simulink model "Project_sim"  (R2025b)
settings: Solver=ode4  StartTime=0.0  StopTime=2*T  FixedStep=0.1  RelTol=1e-3
values from neighbouring files (symbols this model uses):
  a = 3000+R_E    [RUN_ME.m]
  A_0 = [cos(th0+epsilon1) sin(th0+epsilon1) 0; -sin(th0+epsilon1) cos(th0+epsilon1) 0; 0 0 1]*    [1 0 0; 0 cos(i+epsilon2) sin(i+epsilon2); 0 -sin(i+epsilon2) cos(i+epsilon2)]    [RUN_ME.m]
  alpha1 = 0.72    [RUN_ME.m]
  alpha_G0 = 0    [RUN_ME.m]
  AU = astroConstants(2)    [RUN_ME.m]
  b_gyro = deg2rad(0.01*rand(1))    [RUN_ME.m]
  b_mag = 15e-9    (= 1.5e-08)    [RUN_ME.m]
  b_sun = deg2rad(0.1*rand(1))    [RUN_ME.m]
  c_time = 100    [RUN_ME.m]
  D = zeros(3)    [RUN_ME.m]
  den_cz_mag = double(sym2poly(den8_z_mag))    [RUN_ME.m]
  den_cz_sun = double(sym2poly(den8_z_sun))    [RUN_ME.m]
  e = 0.2    [RUN_ME.m]
  epsilon = astroConstants(8)    [RUN_ME.m]
  g_IGRF = [ ... (first row only)    [RUN_ME.m]
  gyro_delay = 1    [RUN_ME.m]
  gyro_mounting = eye(3)    [RUN_ME.m]
  h_IGRF = [ ... (first row only)    [RUN_ME.m]
  I = [Ix 0 0; 0 Iy 0; 0 0 Iz]    [RUN_ME.m]
  i = deg2rad(30)    [RUN_ME.m]
  j_B = [0.01; 0.05; 0.01]    [RUN_ME.m]
  K = place(A, -B, a_controlled)    [RUN_ME.m]
  k1 = 20e-4    (= 0.002)    [RUN_ME.m]
  k1_tilde = 5e-4    (= 0.0005)    [RUN_ME.m]
  k2 = 2e-4    (= 0.0002)    [RUN_ME.m]
  Mis_gyro = deg2rad(0.1*rand(3,1))    [RUN_ME.m]
  Mis_mag = deg2rad(0.1*rand(3,1))    [RUN_ME.m]
  Mis_sun = deg2rad(0.1*rand(3,1))    [RUN_ME.m]
  mu = astroConstants(13)    [RUN_ME.m]
  n = sqrt(mu/a^3)    [RUN_ME.m]
  noise_density_mag = 16e-9    (= 1.6e-08)    [RUN_ME.m]
  Nonorthog_err_gyro = deg2rad(0.1*rand(3,1))    [RUN_ME.m]
  Nonorthog_err_mag = deg2rad(1)*ones(3,1)    [RUN_ME.m]
  num_cz_mag = double(sym2poly(num8_z_mag))    [RUN_ME.m]
  num_cz_sun = double(sym2poly(num8_z_sun))    [RUN_ME.m]
  R_E = astroConstants(23)    [RUN_ME.m]
  R_sun = astroConstants(3)    [RUN_ME.m]
  saturation_gyro = deg2rad(100)    [RUN_ME.m]
  saturation_mag = 60e-6    (= 6e-05)    [RUN_ME.m]
  SF = deg2rad(20*5.25e-3)    [RUN_ME.m]
  SFn = 0.02/100    (= 0.0002)    [RUN_ME.m]
  sigma_ARW = ARW/sqrt(Ts_gyro)    [RUN_ME.m]
  sigma_bias = bias_instability/sqrt(Ts_gyro)    [RUN_ME.m]
  sigma_RRW = RRW/sqrt(Ts_gyro)    [RUN_ME.m]
  sigma_sun = deg2rad(0.5)    [RUN_ME.m]
  th0 = deg2rad(0)    [RUN_ME.m]
  Ts = 0.1    [RUN_ME.m]
  Ts_gyro = 0.1    [RUN_ME.m]
  Ts_mag = 0.1    [RUN_ME.m]
  Ts_sun = 0.1    [RUN_ME.m]
  w_E = 2*pi/T_E    [RUN_ME.m]
  wx_0 = rand(1)*pi/6    [RUN_ME.m]
  wy_0 = rand(1)*pi/6    [RUN_ME.m]
  wz_0 = rand(1)*pi/6    [RUN_ME.m]
undefined symbols (not defined in the file or in its folder): DiscIntNeverNeededParam, dspblkCoreblockFVToolHelper, gcbh, magnitude, precision_sun, RW
libraries: Lib_rotation_matrix x17, matrix_library x11, simulink x3
(part 2 of 3)

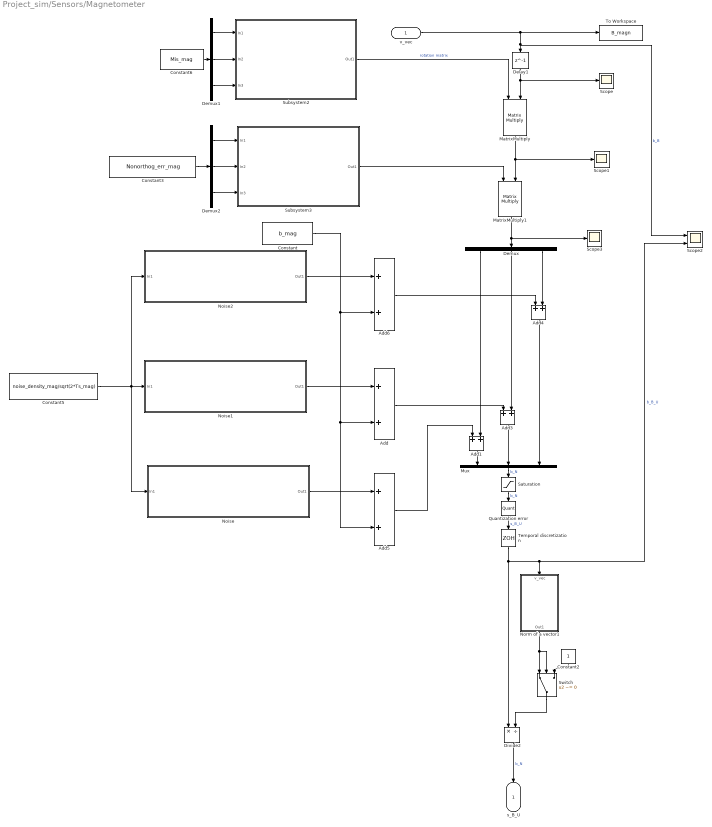
== system Project_sim/Sensors/Magnetometer ==
  v_vec : Inport
  Add{,1,3..6} (6 alike) : Sum
  Constant : Constant  Value=b_mag
  Constant2 : Constant
  Constant3 : Constant  Value=Nonorthog_err_mag
  Constant5 : Constant  Value=noise_density_mag/sqrt(2*Ts_mag)
  Constant6 : Constant  Value=Mis_mag
  Delay1 : Delay  DelayLength=1
  Demux : Demux  Outputs=3
  Demux1 : Demux  Outputs=3
  Demux2 : Demux  Outputs=3
  Divide2 : Product  Inputs=*/
  MatrixMultiply : Product  Multiplication=Matrix(*)
  MatrixMultiply1 : Product  Multiplication=Matrix(*)
  Mux : Mux  Inputs=3
  Noise : Subsystem
  Noise1 : Subsystem
  Noise2 : Subsystem
  Norm of a vector1 : Subsystem
  Quantization error : Quantizer  QuantizationInterval=precision_mag
  Saturation : Saturate  UpperLimit=saturation_mag  LowerLimit=-saturation_mag
  Scope : Scope
      settings: DataLoggingVariableName=ScopeData11  DataLoggingSaveFormat=Array
  Scope1 : Scope
      settings: DataLoggingVariableName=ScopeData13  DataLoggingSaveFormat=Array
  Scope2 : Scope  NumInputPorts=2
      settings: DataLoggingVariableName=ScopeData12  DataLoggingSaveFormat=Array
  Scope3 : Scope
      settings: DataLoggingVariableName=ScopeData15  DataLoggingSaveFormat=Array
  Subsystem2 : Subsystem
  Subsystem3 : Subsystem
  Switch : Switch  Criteria=u2 ~= 0  SaturateOnIntegerOverflow=off  InputSameDT=off
  Temporal discretization : ZeroOrderHold  SampleTime=Ts_mag
  To Workspace : ToWorkspace  VariableName=B_magn  SampleTime=-1
  s_B_U : Outport
  wires:
  v_vec/1 -> Scope2/1, Delay1/1, To Workspace/1  "b_B"
  Subsystem2/1(Out1) -> MatrixMultiply/1  "rotation matrix"
  Norm of a vector1/1(Out1) -> Switch/2, Switch/1
  Demux/1 -> Add1/2
  Demux/2 -> Add3/2
  Demux/3 -> Add4/2
  Add1/1 -> Mux/1
  Add3/1 -> Mux/2
  Add4/1 -> Mux/3
  Constant5/1 -> Noise2/1(In1), Noise/1(In1), Noise1/1(In1)
  Noise/1(Out1) -> Add5/1
  Noise1/1(Out1) -> Add/1
  Noise2/1(Out1) -> Add6/1
  Constant/1 -> Add5/2, Add/2, Add6/2
  Add6/1 -> Add4/1
  Add/1 -> Add3/1
  Add5/1 -> Add1/1
  Demux1/2 -> Subsystem2/2(In2)
  Constant6/1 -> Demux1/1
  Demux1/3 -> Subsystem2/3(In3)
  Demux1/1 -> Subsystem2/1(In1)
  Demux2/2 -> Subsystem3/2(In2)
  Constant3/1 -> Demux2/1
  Demux2/3 -> Subsystem3/3(In3)
  Subsystem3/1(Out1) -> MatrixMultiply1/1
  Demux2/1 -> Subsystem3/1(In1)
  Divide2/1 -> s_B_U/1  "b_N"
  Mux/1 -> Saturation/1  "b_N"
  Saturation/1 -> Quantization error/1  "b_N"
  Switch/1 -> Divide2/2
  Constant2/1 -> Switch/3
  Delay1/1 -> Scope/1, MatrixMultiply/2
  MatrixMultiply/1 -> Scope1/1, MatrixMultiply1/2
  MatrixMultiply1/1 -> Scope3/1, Demux/1
  Quantization error/1 -> Temporal discretization/1  "s_B_U"
  Temporal discretization/1 -> Scope2/2, Norm of a vector1/1(v_vec), Divide2/1  "b_B_U"

== system Project_sim/Sensors/Sun sensor ==
  In1 : Inport
  Enable : EnablePort  StatesWhenEnabling=reset
  Add1 : Sum
  Add3 : Sum
  Add4 : Sum
  Constant : Constant  Value=b_sun
  Constant1 : Constant  Value=Mis_sun
  Constant2 : Constant  Value=sigma_sun
  Delay1 : Delay  DelayLength=1
  Demux : Demux  Outputs=3
  Matrix Multiply1 : Product  Multiplication=Matrix(*)
  Matrix Multiply2 : Product  Multiplication=Matrix(*)
  Noise : Subsystem
  Noise1 : Subsystem
  Noise2 : Subsystem
  Precision : Subsystem  Commented=on
  Scope : Scope
      settings: DataLoggingVariableName=ScopeData6  DataLoggingSaveFormat=Array
  Subsystem1 : Subsystem
  Subsystem2 : Subsystem
  Temporal discretization : ZeroOrderHold  SampleTime=Ts_sun
  s_B_U : Outport  OutputWhenDisabled=reset  InitialOutput=-2
  wires:
  Temporal discretization/1 -> Scope/1, s_B_U/1  "s_B_U"
  In1/1 -> Delay1/1  "s_B"
  Subsystem1/1(Out1) -> Matrix Multiply1/1
  Subsystem2/1(Out1) -> Matrix Multiply2/1
  Matrix Multiply2/1 -> Matrix Multiply1/2
  Noise/1(Out1) -> Add1/2
  Constant1/1 -> Demux/1
  Demux/1 -> Subsystem2/1(In1)
  Demux/3 -> Subsystem2/3(In3)
  Demux/2 -> Subsystem2/2(In2)
  Noise1/1(Out1) -> Add3/2
  Add3/1 -> Subsystem1/3(In3)  "scale factor"
  Noise2/1(Out1) -> Add4/2
  Constant2/1 -> Noise1/1(In1), Noise/1(In1), Noise2/1(In1)
  Constant/1 -> Add3/1, Add1/1, Add4/1
  Add1/1 -> Subsystem1/2(In2)  "scale factor"
  Add4/1 -> Subsystem1/1(In1)  "scale factor"
  Delay1/1 -> Matrix Multiply2/2
  Matrix Multiply1/1 -> Temporal discretization/1

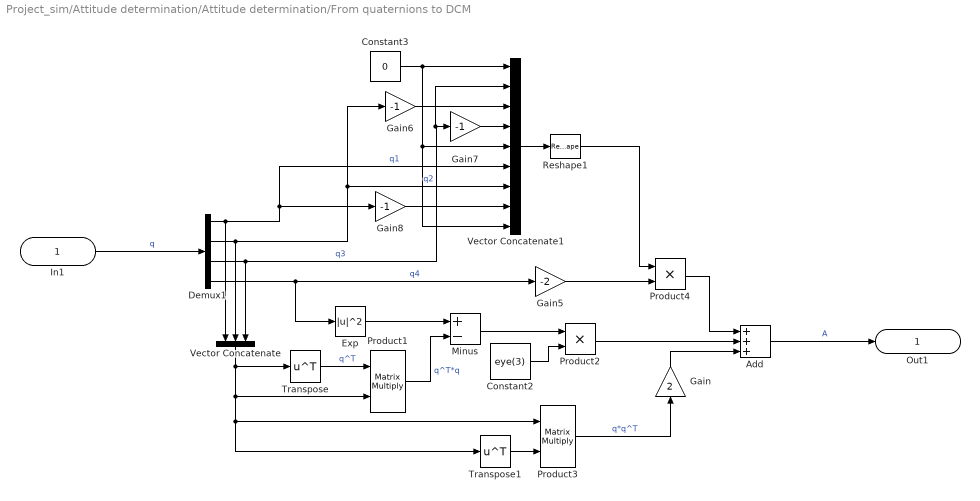
== system Project_sim/Attitude determination/Attitude determination/From quaternions to DCM ==
  In1 : Inport
  Add : Sum  Inputs=+++
  Constant2 : Constant  Value=eye(3)
  Constant3 : Constant  Value=0
  Demux1 : Demux
  Exp : Math  Operator=magnitude^2
  Gain : Gain  Gain=2
  Gain5 : Gain  Gain=-2
  Gain6 : Gain  Gain=-1
  Gain7 : Gain  Gain=-1
  Gain8 : Gain  Gain=-1
  Minus : Sum  Inputs=+-
  Product1 : Product  Multiplication=Matrix(*)
  Product2 : Product
  Product3 : Product  Multiplication=Matrix(*)
  Product4 : Product
  Reshape1 : Reshape  OutputDimensionality=Customize  OutputDimensions=[3,3]
  Transpose : Math  Operator=transpose
  Transpose1 : Math  Operator=transpose
  Vector Concatenate : Concatenate  NumInputs=3
  Vector Concatenate1 : Concatenate  NumInputs=9
  Out1 : Outport
  wires:
  Constant2/1 -> Product2/2
  Transpose1/1 -> Product3/2
  Exp/1 -> Minus/1
  Product2/1 -> Add/2
  Vector Concatenate/1 -> Product1/2, Product3/1, Transpose1/1, Transpose/1
  Transpose/1 -> Product1/1  "q^T"
  Gain/1 -> Add/3
  Add/1 -> Out1/1  "A"
  Demux1/4 -> Exp/1, Gain5/1  "q4"
  Demux1/1 -> Vector Concatenate/1, Gain8/1, Vector Concatenate1/6  "q1"
  Vector Concatenate1/1 -> Reshape1/1
  Product1/1 -> Minus/2  "q^T*q"
  Gain5/1 -> Product4/2
  In1/1 -> Demux1/1  "q"
  Minus/1 -> Product2/1
  Demux1/2 -> Vector Concatenate1/7, Gain6/1, Vector Concatenate/2  "q2"
  Gain8/1 -> Vector Concatenate1/8
  Product4/1 -> Add/1
  Reshape1/1 -> Product4/1
  Constant3/1 -> Vector Concatenate1/9, Vector Concatenate1/5, Vector Concatenate1/1
  Demux1/3 -> Vector Concatenate1/2, Gain7/1, Vector Concatenate/3  "q3"
  Gain6/1 -> Vector Concatenate1/3
  Gain7/1 -> Vector Concatenate1/4
  Product3/1 -> Gain/1  "q*q^T"

== system Project_sim/Attitude determination/Attitude determination/Trace of a matrix ==
  M : Inport
  Add2 : Sum  Inputs=+++
  Demux : Demux  Outputs=9
  Reshape : Reshape  OutputDimensionality=Column vector (2-D)
  tr(M) : Outport
  wires:
  Demux/5 -> Add2/2
  Demux/1 -> Add2/1
  Reshape/1 -> Demux/1
  Demux/9 -> Add2/3
  M/1 -> Reshape/1
  Add2/1 -> tr(M)/1  "tr(M)"

== system Project_sim/Control system/Control Manager/If Action Subsystem ==
  In1 : Inport
  Action Port : ActionPort  InitializeStates=reset  PropagateVarSize=During execution  ActionPortLabel=if(u1<u2 & u3 >100)
  Out1 : Outport
  wires:
  In1/1 -> Out1/1  "1"

== system Project_sim/Control system/Control Manager/If Action Subsystem1 ==
  In1 : Inport
  Action Port : ActionPort  InitializeStates=reset  PropagateVarSize=During execution  ActionPortLabel=if(u1 ==1 & u2 < u3 & u4 <u5 & u6 > 200)
  Out1 : Outport
  wires:
  In1/1 -> Out1/1  "1"

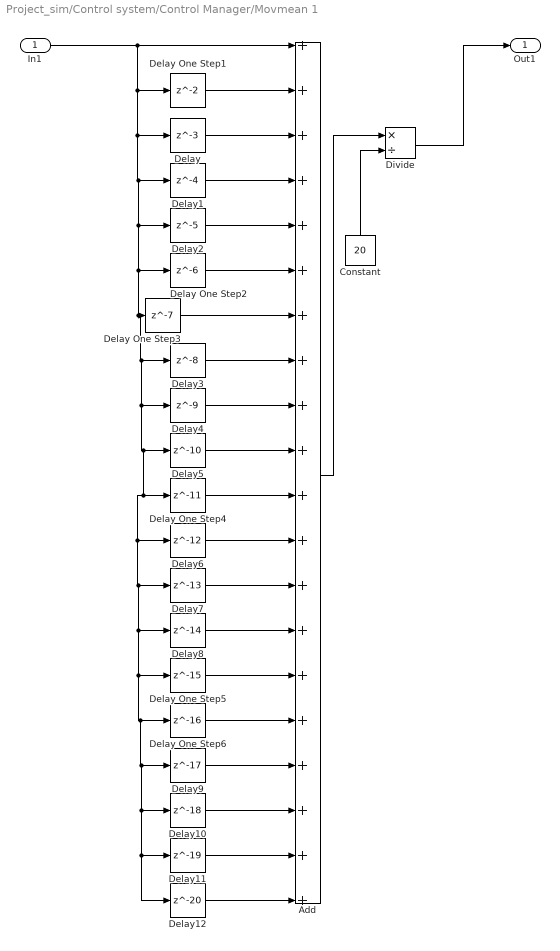
== system Project_sim/Control system/Control Manager/Movmean 1 ==
  In1 : Inport
  Add : Sum  Inputs=++++++++++++++++++++
  Constant : Constant  Value=20
  Delay : Delay  DelayLength=3
  Delay One Step1 : Delay
  Delay One Step2 : Delay  DelayLength=6
  Delay One Step3 : Delay  DelayLength=7
  Delay One Step4 : Delay  DelayLength=11
  Delay One Step5 : Delay  DelayLength=15
  Delay One Step6 : Delay  DelayLength=16
  Delay1 : Delay  DelayLength=4
  Delay10 : Delay  DelayLength=18
  Delay11 : Delay  DelayLength=19
  Delay12 : Delay  DelayLength=20
  Delay2 : Delay  DelayLength=5
  Delay3 : Delay  DelayLength=8
  Delay4 : Delay  DelayLength=9
  Delay5 : Delay  DelayLength=10
  Delay6 : Delay  DelayLength=12
  Delay7 : Delay  DelayLength=13
  Delay8 : Delay  DelayLength=14
  Delay9 : Delay  DelayLength=17
  Divide : Product  Inputs=*/
  Out1 : Outport
  wires:
  Delay One Step1/1 -> Add/2
  Delay/1 -> Add/3
  Delay1/1 -> Add/4
  Delay2/1 -> Add/5
  Add/1 -> Divide/1
  Constant/1 -> Divide/2
  Divide/1 -> Out1/1
  Delay One Step2/1 -> Add/6
  Delay One Step3/1 -> Add/7
  Delay3/1 -> Add/8
  Delay4/1 -> Add/9
  Delay5/1 -> Add/10
  Delay One Step6/1 -> Add/16
  Delay6/1 -> Add/12
  Delay10/1 -> Add/18
  Delay11/1 -> Add/19
  Delay One Step5/1 -> Add/15
  Delay7/1 -> Add/13
  Delay9/1 -> Add/17
  Delay8/1 -> Add/14
  In1/1 -> Delay2/1, Delay One Step2/1, Delay8/1, Delay One Step5/1, Delay12/1, Delay11/1, Delay10/1, Delay9/1, Delay One Step6/1, Delay7/1, Delay6/1, Delay One Step4/1, Delay5/1, Delay4/1, Delay3/1, Delay One Step3/1, Delay1/1, Delay/1, Delay One Step1/1, Add/1
  Delay One Step4/1 -> Add/11
  Delay12/1 -> Add/20

== system Project_sim/Control system/Control Manager/Movmean 2 ==
  In1 : Inport
  Add : Sum  Inputs=++++++++++
  Constant : Constant  Value=10
  Delay : Delay  DelayLength=3
  Delay One Step1 : Delay
  Delay One Step2 : Delay  DelayLength=6
  Delay One Step3 : Delay  DelayLength=7
  Delay1 : Delay  DelayLength=4
  Delay2 : Delay  DelayLength=5
  Delay3 : Delay  DelayLength=8
  Delay4 : Delay  DelayLength=9
  Delay5 : Delay  DelayLength=10
  Divide : Product  Inputs=*/
  Out1 : Outport
  wires:
  Delay One Step1/1 -> Add/2
  In1/1 -> Add/1, Delay2/1, Delay5/1, Delay4/1, Delay3/1, Delay One Step3/1, Delay One Step2/1, Delay1/1, Delay/1, Delay One Step1/1
  Delay/1 -> Add/3
  Delay1/1 -> Add/4
  Delay2/1 -> Add/5
  Add/1 -> Divide/1
  Constant/1 -> Divide/2
  Divide/1 -> Out1/1
  Delay One Step2/1 -> Add/6
  Delay One Step3/1 -> Add/7
  Delay3/1 -> Add/8
  Delay4/1 -> Add/9
  Delay5/1 -> Add/10

== system Project_sim/Control system/Control Manager/Movmean 3 ==
  In1 : Inport
  Add : Sum  Inputs=++++++++++
  Constant : Constant  Value=10
  Delay : Delay  DelayLength=3
  Delay One Step1 : Delay
  Delay One Step2 : Delay  DelayLength=6
  Delay One Step3 : Delay  DelayLength=7
  Delay1 : Delay  DelayLength=4
  Delay2 : Delay  DelayLength=5
  Delay3 : Delay  DelayLength=8
  Delay4 : Delay  DelayLength=9
  Delay5 : Delay  DelayLength=10
  Divide : Product  Inputs=*/
  Out1 : Outport
  wires:
  Delay One Step1/1 -> Add/2
  In1/1 -> Add/1, Delay2/1, Delay5/1, Delay4/1, Delay3/1, Delay One Step3/1, Delay One Step2/1, Delay1/1, Delay/1, Delay One Step1/1
  Delay/1 -> Add/3
  Delay1/1 -> Add/4
  Delay2/1 -> Add/5
  Add/1 -> Divide/1
  Constant/1 -> Divide/2
  Divide/1 -> Out1/1
  Delay One Step2/1 -> Add/6
  Delay One Step3/1 -> Add/7
  Delay3/1 -> Add/8
  Delay4/1 -> Add/9
  Delay5/1 -> Add/10

== system Project_sim/Control system/Control Manager/Norm of a vector1 ==
  v_vec : Inport
  Add : Sum  Inputs=+++
  Demux : Demux  Outputs=3
  Magnitude Squared : Math  Operator=magnitude^2
  Magnitude Squared1 : Math  Operator=magnitude^2
  Magnitude Squared2 : Math  Operator=magnitude^2
  Square Root : Sqrt
  Out1 : Outport
  wires:
  Square Root/1 -> Out1/1  "norm(v)"
  Magnitude Squared2/1 -> Add/3
  Demux/3 -> Magnitude Squared2/1
  Add/1 -> Square Root/1
  Demux/1 -> Magnitude Squared/1
  Magnitude Squared/1 -> Add/1
  Magnitude Squared1/1 -> Add/2
  Demux/2 -> Magnitude Squared1/1
  v_vec/1 -> Demux/1  "v_vec"

== system Project_sim/Control system/Control Manager/Norm of a vector2 ==
  v_vec : Inport
  Add : Sum  Inputs=+++
  Demux : Demux  Outputs=3
  Magnitude Squared : Math  Operator=magnitude^2
  Magnitude Squared1 : Math  Operator=magnitude^2
  Magnitude Squared2 : Math  Operator=magnitude^2
  Square Root : Sqrt
  Out1 : Outport
  wires:
  Square Root/1 -> Out1/1  "norm(v)"
  Magnitude Squared2/1 -> Add/3
  Demux/3 -> Magnitude Squared2/1
  Add/1 -> Square Root/1
  Demux/1 -> Magnitude Squared/1
  Magnitude Squared/1 -> Add/1
  Magnitude Squared1/1 -> Add/2
  Demux/2 -> Magnitude Squared1/1
  v_vec/1 -> Demux/1  "v_vec"

== system Project_sim/Control system/Control Manager/Norm of a vector3 ==
  v_vec : Inport
  Add : Sum  Inputs=+++
  Demux : Demux  Outputs=3
  Magnitude Squared : Math  Operator=magnitude^2
  Magnitude Squared1 : Math  Operator=magnitude^2
  Magnitude Squared2 : Math  Operator=magnitude^2
  Square Root : Sqrt
  Out1 : Outport
  Out2 : Outport  Port=2
  wires:
  Square Root/1 -> Out1/1  "norm(v)"
  Magnitude Squared2/1 -> Add/3
  Demux/3 -> Magnitude Squared2/1
  Add/1 -> Square Root/1
  Demux/1 -> Magnitude Squared/1
  Magnitude Squared/1 -> Add/1
  Magnitude Squared1/1 -> Add/2
  Demux/2 -> Magnitude Squared1/1
  v_vec/1 -> Demux/1  "v_vec"

== system Project_sim/Disturbances/Gravity Gradient/Norm of a vector ==
  v_vec : Inport
  Add : Sum  Inputs=+++
  Demux : Demux  Outputs=3
  Magnitude Squared : Math  Operator=magnitude^2
  Magnitude Squared1 : Math  Operator=magnitude^2
  Magnitude Squared2 : Math  Operator=magnitude^2
  Square Root : Sqrt
  Out1 : Outport
  wires:
  Square Root/1 -> Out1/1  "norm(v)"
  Magnitude Squared2/1 -> Add/3
  Demux/3 -> Magnitude Squared2/1
  Add/1 -> Square Root/1
  Demux/1 -> Magnitude Squared/1
  Magnitude Squared/1 -> Add/1
  Magnitude Squared1/1 -> Add/2
  Demux/2 -> Magnitude Squared1/1
  v_vec/1 -> Demux/1  "v_vec"

== system Project_sim/Environment/Eclipse Simulation/dist_sat_2_phi ==
  dist_sat : Inport
  z_sat : Inport  Port=2
  Constant : Constant  Value=0
  Constant5 : Constant
  Max : MinMax  Function=max  Inputs=2
  Subtract1 : Sum  Inputs=+-
  sin_phi^2 : Math  Operator=square
  sqrt2 : Sqrt
  sum76 : Product  Inputs=/*
  sin_phi : Outport
  cos_phi : Outport  Port=2
  wires:
  Constant5/1 -> Subtract1/1
  dist_sat/1 -> sum76/1
  sin_phi^2/1 -> Subtract1/2
  Constant/1 -> Max/2
  Max/1 -> sqrt2/1
  sum76/1 -> sin_phi/1, sin_phi^2/1
  Subtract1/1 -> Max/1
  sqrt2/1 -> cos_phi/1
  z_sat/1 -> sum76/2

== system Project_sim/Environment/Eclipse Simulation/phi_R_E_2_R_EARTH_LOC ==
  sin_phi : Inport
  cos_phi : Inport  Port=2
  R_POL : Inport  Port=3
  R_EQ : Inport  Port=4
  Divide : Product  Inputs=*/
  Product{,1..3} (4 alike) : Product
  Square{3..8} (6 alike) : Math  Operator=square
  den : Sum
  num : Sum
  sqrt768 : Sqrt
  R_EARTH_LOC : Outport
  wires:
  Square3/1 -> Product/2
  Square7/1 -> den/1
  Square6/1 -> num/2
  sin_phi/1 -> Product1/1, Product3/1
  den/1 -> Divide/2
  cos_phi/1 -> Product2/1, Product/1
  Divide/1 -> sqrt768/1
  R_EQ/1 -> Square3/1, Product2/2
  Square8/1 -> den/2
  Square5/1 -> num/1
  R_POL/1 -> Square4/1, Product3/2
  Product2/1 -> Square8/1
  Product3/1 -> Square7/1
  num/1 -> Divide/1
  Product/1 -> Square6/1
  Square4/1 -> Product1/2
  Product1/1 -> Square5/1
  sqrt768/1 -> R_EARTH_LOC/1

== system Project_sim/Environment/Eclipse Simulation/r_sat_2_dist_sat ==
  r_sat : Inport
  Square : Math  Operator=square
  Square1 : Math  Operator=square
  Square2 : Math  Operator=square
  "r_sat(1), r_sat(2), r_sat(3)" : Demux  Outputs=3
  r_sq : Sum  Inputs=+++
  sqrt1 : Sqrt
  dist_sat : Outport
  z_sat : Outport  Port=2
  wires:
  Square1/1 -> r_sq/2
  "r_sat(1), r_sat(2), r_sat(3)"/2 -> Square1/1  "y_sat"
  "r_sat(1), r_sat(2), r_sat(3)"/3 -> z_sat/1, Square2/1  "z_sat"
  "r_sat(1), r_sat(2), r_sat(3)"/1 -> Square/1  "x_sat"
  r_sq/1 -> sqrt1/1
  Square/1 -> r_sq/1
  Square2/1 -> r_sq/3
  sqrt1/1 -> dist_sat/1
  r_sat/1 -> "r_sat(1), r_sat(2), r_sat(3)"/1

== system Project_sim/Environment/Eclipse Simulation/r_sat_sun_2_dist_sat_sun ==
  r_sat_sun : Inport
  Square10 : Math  Operator=square
  Square11 : Math  Operator=square
  Square9 : Math  Operator=square
  "r_sat_sun(1), r_sat_sun(2), r_sat_sun(3)" : Demux  Outputs=3
  r_sat_sun_sq : Sum  Inputs=+++
  sqrt54 : Sqrt
  dist_sat_sun : Outport
  wires:
  "r_sat_sun(1), r_sat_sun(2), r_sat_sun(3)"/2 -> Square10/1  "y_sat_sun"
  Square11/1 -> r_sat_sun_sq/3
  Square10/1 -> r_sat_sun_sq/2
  Square9/1 -> r_sat_sun_sq/1
  r_sat_sun_sq/1 -> sqrt54/1
  "r_sat_sun(1), r_sat_sun(2), r_sat_sun(3)"/1 -> Square9/1  "x_sat_sun"
  "r_sat_sun(1), r_sat_sun(2), r_sat_sun(3)"/3 -> Square11/1  "z_sat_sun"
  r_sat_sun/1 -> "r_sat_sun(1), r_sat_sun(2), r_sat_sun(3)"/1
  sqrt54/1 -> dist_sat_sun/1

== system Project_sim/Reaction Wheels/Omit sample until settling time/If Action Subsystem ==
  Action Port : ActionPort  ActionPortLabel=if(u1 <= Ts)
  Zero : Constant  Value=0  OutDataTypeStr=Inherit: Inherit via back propagation
  Out1 : Outport
  wires:
  Zero/1 -> Out1/1

== system Project_sim/Reaction Wheels/Omit sample until settling time/If Action Subsystem1 ==
  Action Port : ActionPort  ActionPortLabel=else
  One : Constant  OutDataTypeStr=Inherit: Inherit via back propagation
  Out1 : Outport
  wires:
  One/1 -> Out1/1

== system Project_sim/Reaction Wheels/Saturation/Max_torque(omega) ==
  omega_RW : Inport
  Constant : Constant  Value=RW.max_torque_start_descending
  If : If  NumInputs=2  IfExpression=u2 <= u1 & u2 >= -u1
  If Action Subsystem : Subsystem  TreatAsAtomicUnit=on
  If Action Subsystem1 : Subsystem  TreatAsAtomicUnit=on
  Merge : Merge
  M_max : Outport
  wires:
  If Action Subsystem/1(Out1) -> Merge/1
  If/2 -> If Action Subsystem1/Action
  If Action Subsystem1/1(Out1) -> Merge/2
  omega_RW/1 -> If Action Subsystem1/1(In1), If/2  "omega_RW"
  Merge/1 -> M_max/1
  If/1 -> If Action Subsystem/Action
  Constant/1 -> If/1

== system Project_sim/Reaction Wheels/Saturation/Max_torque(omega)1 ==
  omega_RW : Inport
  Constant : Constant  Value=RW.max_torque_start_descending
  If : If  NumInputs=2  IfExpression=u2 <= u1 & u2 >= -u1
  If Action Subsystem : Subsystem  TreatAsAtomicUnit=on
  If Action Subsystem1 : Subsystem  TreatAsAtomicUnit=on
  Merge : Merge
  M_max : Outport
  wires:
  If Action Subsystem/1(Out1) -> Merge/1
  If/2 -> If Action Subsystem1/Action
  If Action Subsystem1/1(Out1) -> Merge/2
  omega_RW/1 -> If Action Subsystem1/1(In1), If/2  "omega_RW"
  Merge/1 -> M_max/1
  If/1 -> If Action Subsystem/Action
  Constant/1 -> If/1

== system Project_sim/Reaction Wheels/Saturation/Max_torque(omega)2 ==
  omega_RW : Inport
  Constant : Constant  Value=RW.max_torque_start_descending
  If : If  NumInputs=2  IfExpression=u2 <= u1 & u2 >= -u1
  If Action Subsystem : Subsystem  TreatAsAtomicUnit=on
  If Action Subsystem1 : Subsystem  TreatAsAtomicUnit=on
  Merge : Merge
  M_max : Outport
  wires:
  If Action Subsystem/1(Out1) -> Merge/1
  If/2 -> If Action Subsystem1/Action
  If Action Subsystem1/1(Out1) -> Merge/2
  omega_RW/1 -> If Action Subsystem1/1(In1), If/2  "omega_RW"
  Merge/1 -> M_max/1
  If/1 -> If Action Subsystem/Action
  Constant/1 -> If/1

== system Project_sim/Sensors/Gyroscope/Noise manager ==
  Add : Sum  Inputs=+++
  Discrete Transfer Fcn1 : DiscreteTransferFcn  LoadFcn=dspblkCoreblockFVToolHelper(gcbh,'load');  Numerator=num_cz_sun  Denominator=den_cz_sun
      settings: CopyFcn=dspblkCoreblockFVToolHelper(gcbh,'copy');  DeleteFcn=dspblkCoreblockFVToolHelper(gcbh,'close');  ModelCloseFcn=dspblkCoreblockFVToolHelper(gcbh,'close');  PreSaveFcn=dspblkCoreblockFVToolHelper(gcbh,'presave');  PostSaveFcn=dspblkCoreblockFVToolHelper(gcbh,'postsave');  CloseFcn=dspblkCoreblockFVToolHelper(gcbh,'close');
  Discrete-Time Integrator : DiscreteIntegrator  SampleTime=Ts_gyro  ICPrevOutput=DiscIntNeverNeededParam  ICPrevScaledInput=DiscIntNeverNeededParam
  Gain : Gain  Gain=sigma_bias
  Gain1 : Gain  Gain=sigma_RRW
  Gain2 : Gain  Gain=sigma_ARW
  Gain3 : Gain  Gain=1/c_time
  Random Number : RandomNumber  Seed=randi(1e6)  SampleTime=Ts_gyro
  Random Number4 : RandomNumber  Seed=randi(1e6)  SampleTime=Ts_gyro
  Random Number5 : RandomNumber  Seed=randi(1e6)  SampleTime=Ts_gyro
  Sum : Sum  Inputs=-+|
  Out1 : Outport
  wires:
  Gain1/1 -> Discrete Transfer Fcn1/1
  Gain2/1 -> Add/3  "angle walk error"
  Discrete-Time Integrator/1 -> Gain3/1, Add/1  "bias instability"
  Discrete Transfer Fcn1/1 -> Add/2  "random walk error"
  Random Number/1 -> Gain/1
  Add/1 -> Out1/1  "noise"
  Random Number4/1 -> Gain1/1
  Random Number5/1 -> Gain2/1
  Gain3/1 -> Sum/1
  Sum/1 -> Discrete-Time Integrator/1
  Gain/1 -> Sum/2

== system Project_sim/Sensors/Gyroscope/Subsystem2 ==
  In1 : Inport
  In2 : Inport  Port=2
  In3 : Inport  Port=3
  A1 : Lib_rotation_matrix/A1  SystemSampleTime=-1  VariantActivationTime=update diagram  EmptyChoice=off  PassThrough=off  PassThroughVariantControl=(default)  EmptyChoiceVariantControl=(default)  AllowFlexibleInterface=on  Latency=0  AutoFrameSizeCalculation=off
  A2 : Lib_rotation_matrix/A2  SystemSampleTime=-1  VariantActivationTime=update diagram  EmptyChoice=off  PassThrough=off  PassThroughVariantControl=(default)  EmptyChoiceVariantControl=(default)  AllowFlexibleInterface=on  Latency=0  AutoFrameSizeCalculation=off
  A3 : Lib_rotation_matrix/A3  SystemSampleTime=-1  VariantActivationTime=update diagram  EmptyChoice=off  PassThrough=off  PassThroughVariantControl=(default)  EmptyChoiceVariantControl=(default)  AllowFlexibleInterface=on  Latency=0  AutoFrameSizeCalculation=off
  MatrixMultiply : Product  Multiplication=Matrix(*)
  MatrixMultiply1 : Product  Multiplication=Matrix(*)
  Out1 : Outport
  wires:
  MatrixMultiply/1 -> MatrixMultiply1/1
  A3/1 -> MatrixMultiply1/2
  A1/1 -> MatrixMultiply/1
  MatrixMultiply1/1 -> Out1/1  "rotation matrix"
  A2/1 -> MatrixMultiply/2
  In1/1 -> A1/1  "amplitude of misalignment x"
  In2/1 -> A2/1  "amplitude of misalignment y"
  In3/1 -> A3/1  "amplitude of misalignment z"

== system Project_sim/Sensors/Gyroscope/Subsystem3 ==
  In1 : Inport
  In2 : Inport  Port=2
  In3 : Inport  Port=3
  MatrixMultiply1 : Product  Multiplication=Matrix(*)
  One : Constant  OutDataTypeStr=Inherit: Inherit via back propagation
  Reshape : Reshape  OutputDimensionality=Customize  OutputDimensions=[3,3]
  Reshape1 : Reshape  OutputDimensionality=Customize  OutputDimensions=[3,3]
  Vector Concatenate : Concatenate  NumInputs=9
  Vector Concatenate1 : Concatenate  NumInputs=9
  Zero : Constant  Value=0  OutDataTypeStr=Inherit: Inherit via back propagation
  Out1 : Outport
  wires:
  Reshape/1 -> MatrixMultiply1/1
  MatrixMultiply1/1 -> Out1/1  "rotation matrix"
  In1/1 -> Vector Concatenate1/4, Vector Concatenate1/2, Vector Concatenate/2  "amplitude of nonrothog 1"
  In2/1 -> Vector Concatenate/3, Vector Concatenate1/7, Vector Concatenate1/3  "amplitude of nonrothog 2"
  In3/1 -> Vector Concatenate1/8, Vector Concatenate1/6, Vector Concatenate/6  "amplitude of nonrothog 3"
  Vector Concatenate/1 -> Reshape/1
  Vector Concatenate1/1 -> Reshape1/1
  One/1 -> Vector Concatenate/5, Vector Concatenate/9, Vector Concatenate1/1, Vector Concatenate1/5, Vector Concatenate1/9, Vector Concatenate/1
  Zero/1 -> Vector Concatenate/8, Vector Concatenate/7, Vector Concatenate/4
  Reshape1/1 -> MatrixMultiply1/2

== system Project_sim/Sensors/Magnetometer/Noise ==
  In1 : Inport
  Add6 : Sum  Inputs=+++
  Discrete Transfer Fcn : DiscreteTransferFcn  LoadFcn=dspblkCoreblockFVToolHelper(gcbh,'load');  Numerator=[0.001*Ts_mag 0.001*Ts_mag]  Denominator=[2+0.001*Ts_mag 0.001*Ts_mag-2]
      settings: CopyFcn=dspblkCoreblockFVToolHelper(gcbh,'copy');  DeleteFcn=dspblkCoreblockFVToolHelper(gcbh,'close');  ModelCloseFcn=dspblkCoreblockFVToolHelper(gcbh,'close');  PreSaveFcn=dspblkCoreblockFVToolHelper(gcbh,'presave');  PostSaveFcn=dspblkCoreblockFVToolHelper(gcbh,'postsave');  CloseFcn=dspblkCoreblockFVToolHelper(gcbh,'close');
  Discrete Transfer Fcn5 : DiscreteTransferFcn  LoadFcn=dspblkCoreblockFVToolHelper(gcbh,'load');  Numerator=num_cz_mag  Denominator=den_cz_mag
      settings: CopyFcn=dspblkCoreblockFVToolHelper(gcbh,'copy');  DeleteFcn=dspblkCoreblockFVToolHelper(gcbh,'close');  ModelCloseFcn=dspblkCoreblockFVToolHelper(gcbh,'close');  PreSaveFcn=dspblkCoreblockFVToolHelper(gcbh,'presave');  PostSaveFcn=dspblkCoreblockFVToolHelper(gcbh,'postsave');  CloseFcn=dspblkCoreblockFVToolHelper(gcbh,'close');
  Product : Product
  Product1 : Product
  Product2 : Product
  Random Number6 : RandomNumber  Seed=randi(1e6)  SampleTime=Ts_mag
  Random Number7 : RandomNumber  Seed=randi(1e6)  SampleTime=Ts_mag
  Random Number8 : RandomNumber  Seed=randi(1e6)  SampleTime=Ts_mag
  Out1 : Outport
  wires:
  Random Number7/1 -> Product1/2
  Discrete Transfer Fcn5/1 -> Add6/2  "pink noise"
  Product1/1 -> Discrete Transfer Fcn5/1
  Discrete Transfer Fcn/1 -> Add6/1  "brown noise"
  Product/1 -> Discrete Transfer Fcn/1
  Product2/1 -> Add6/3  "white noise"
  Random Number6/1 -> Product2/2
  Random Number8/1 -> Product/2
  Add6/1 -> Out1/1  "noise"
  In1/1 -> Product2/1, Product1/1, Product/1  "sigma"

== system Project_sim/Sensors/Magnetometer/Noise1 ==
  In1 : Inport
  Add6 : Sum  Inputs=+++
  Discrete Transfer Fcn : DiscreteTransferFcn  LoadFcn=dspblkCoreblockFVToolHelper(gcbh,'load');  Numerator=[0.001*Ts_mag 0.001*Ts_mag]  Denominator=[2+0.001*Ts_mag 0.001*Ts_mag-2]
      settings: CopyFcn=dspblkCoreblockFVToolHelper(gcbh,'copy');  DeleteFcn=dspblkCoreblockFVToolHelper(gcbh,'close');  ModelCloseFcn=dspblkCoreblockFVToolHelper(gcbh,'close');  PreSaveFcn=dspblkCoreblockFVToolHelper(gcbh,'presave');  PostSaveFcn=dspblkCoreblockFVToolHelper(gcbh,'postsave');  CloseFcn=dspblkCoreblockFVToolHelper(gcbh,'close');
  Discrete Transfer Fcn5 : DiscreteTransferFcn  LoadFcn=dspblkCoreblockFVToolHelper(gcbh,'load');  Numerator=num_cz_mag  Denominator=den_cz_mag
      settings: CopyFcn=dspblkCoreblockFVToolHelper(gcbh,'copy');  DeleteFcn=dspblkCoreblockFVToolHelper(gcbh,'close');  ModelCloseFcn=dspblkCoreblockFVToolHelper(gcbh,'close');  PreSaveFcn=dspblkCoreblockFVToolHelper(gcbh,'presave');  PostSaveFcn=dspblkCoreblockFVToolHelper(gcbh,'postsave');  CloseFcn=dspblkCoreblockFVToolHelper(gcbh,'close');
  Product : Product
  Product1 : Product
  Product2 : Product
  Random Number6 : RandomNumber  Seed=randi(1e6)  SampleTime=Ts_mag
  Random Number7 : RandomNumber  Seed=randi(1e6)  SampleTime=Ts_mag
  Random Number8 : RandomNumber  Seed=randi(1e6)  SampleTime=Ts_mag
  Out1 : Outport
  wires:
  Random Number7/1 -> Product1/2
  Discrete Transfer Fcn5/1 -> Add6/2  "pink noise"
  Product1/1 -> Discrete Transfer Fcn5/1
  Discrete Transfer Fcn/1 -> Add6/1  "brown noise"
  Product/1 -> Discrete Transfer Fcn/1
  Product2/1 -> Add6/3  "white noise"
  Random Number6/1 -> Product2/2
  Random Number8/1 -> Product/2
  Add6/1 -> Out1/1  "noise"
  In1/1 -> Product2/1, Product1/1, Product/1  "sigma"

== system Project_sim/Sensors/Magnetometer/Noise2 ==
  In1 : Inport
  Add6 : Sum  Inputs=+++
  Discrete Transfer Fcn : DiscreteTransferFcn  LoadFcn=dspblkCoreblockFVToolHelper(gcbh,'load');  Numerator=[0.001*Ts_mag 0.001*Ts_mag]  Denominator=[2+0.001*Ts_mag 0.001*Ts_mag-2]
      settings: CopyFcn=dspblkCoreblockFVToolHelper(gcbh,'copy');  DeleteFcn=dspblkCoreblockFVToolHelper(gcbh,'close');  ModelCloseFcn=dspblkCoreblockFVToolHelper(gcbh,'close');  PreSaveFcn=dspblkCoreblockFVToolHelper(gcbh,'presave');  PostSaveFcn=dspblkCoreblockFVToolHelper(gcbh,'postsave');  CloseFcn=dspblkCoreblockFVToolHelper(gcbh,'close');
  Discrete Transfer Fcn5 : DiscreteTransferFcn  LoadFcn=dspblkCoreblockFVToolHelper(gcbh,'load');  Numerator=num_cz_mag  Denominator=den_cz_mag
      settings: CopyFcn=dspblkCoreblockFVToolHelper(gcbh,'copy');  DeleteFcn=dspblkCoreblockFVToolHelper(gcbh,'close');  ModelCloseFcn=dspblkCoreblockFVToolHelper(gcbh,'close');  PreSaveFcn=dspblkCoreblockFVToolHelper(gcbh,'presave');  PostSaveFcn=dspblkCoreblockFVToolHelper(gcbh,'postsave');  CloseFcn=dspblkCoreblockFVToolHelper(gcbh,'close');
  Product : Product
  Product1 : Product
  Product2 : Product
  Random Number6 : RandomNumber  Seed=randi(1e6)  SampleTime=Ts_mag
  Random Number7 : RandomNumber  Seed=randi(1e6)  SampleTime=Ts_mag
  Random Number8 : RandomNumber  Seed=randi(1e6)  SampleTime=Ts_mag
  Out1 : Outport
  wires:
  Random Number7/1 -> Product1/2
  Discrete Transfer Fcn5/1 -> Add6/2  "pink noise"
  Product1/1 -> Discrete Transfer Fcn5/1
  Discrete Transfer Fcn/1 -> Add6/1  "brown noise"
  Product/1 -> Discrete Transfer Fcn/1
  Product2/1 -> Add6/3  "white noise"
  Random Number6/1 -> Product2/2
  Random Number8/1 -> Product/2
  Add6/1 -> Out1/1  "noise"
  In1/1 -> Product2/1, Product1/1, Product/1  "sigma"

== system Project_sim/Sensors/Magnetometer/Norm of a vector1 ==
  v_vec : Inport
  Add : Sum  Inputs=+++
  Demux : Demux  Outputs=3
  Magnitude Squared : Math  Operator=magnitude^2
  Magnitude Squared1 : Math  Operator=magnitude^2
  Magnitude Squared2 : Math  Operator=magnitude^2
  Square Root : Sqrt
  Out1 : Outport
  wires:
  Square Root/1 -> Out1/1  "norm(v)"
  Magnitude Squared2/1 -> Add/3
  Demux/3 -> Magnitude Squared2/1
  Add/1 -> Square Root/1
  Demux/1 -> Magnitude Squared/1
  Magnitude Squared/1 -> Add/1
  Magnitude Squared1/1 -> Add/2
  Demux/2 -> Magnitude Squared1/1
  v_vec/1 -> Demux/1  "v_vec"

== system Project_sim/Sensors/Magnetometer/Subsystem2 ==
  In1 : Inport
  In2 : Inport  Port=2
  In3 : Inport  Port=3
  A1 : Lib_rotation_matrix/A1  SystemSampleTime=-1  VariantActivationTime=update diagram  EmptyChoice=off  PassThrough=off  PassThroughVariantControl=(default)  EmptyChoiceVariantControl=(default)  AllowFlexibleInterface=on  Latency=0  AutoFrameSizeCalculation=off
  A2 : Lib_rotation_matrix/A2  SystemSampleTime=-1  VariantActivationTime=update diagram  EmptyChoice=off  PassThrough=off  PassThroughVariantControl=(default)  EmptyChoiceVariantControl=(default)  AllowFlexibleInterface=on  Latency=0  AutoFrameSizeCalculation=off
  A3 : Lib_rotation_matrix/A3  SystemSampleTime=-1  VariantActivationTime=update diagram  EmptyChoice=off  PassThrough=off  PassThroughVariantControl=(default)  EmptyChoiceVariantControl=(default)  AllowFlexibleInterface=on  Latency=0  AutoFrameSizeCalculation=off
  MatrixMultiply : Product  Multiplication=Matrix(*)
  MatrixMultiply1 : Product  Multiplication=Matrix(*)
  Out1 : Outport
  wires:
  MatrixMultiply/1 -> MatrixMultiply1/1
  A3/1 -> MatrixMultiply1/2
  A1/1 -> MatrixMultiply/1
  MatrixMultiply1/1 -> Out1/1  "rotation matrix"
  A2/1 -> MatrixMultiply/2
  In1/1 -> A1/1  "amplitude of misalignment x"
  In2/1 -> A2/1  "amplitude of misalignment y"
  In3/1 -> A3/1  "amplitude of misalignment z"

== system Project_sim/Sensors/Magnetometer/Subsystem3 ==
  In1 : Inport
  In2 : Inport  Port=2
  In3 : Inport  Port=3
  MatrixMultiply1 : Product  Multiplication=Matrix(*)
  One : Constant  OutDataTypeStr=Inherit: Inherit via back propagation
  Reshape : Reshape  OutputDimensionality=Customize  OutputDimensions=[3,3]
  Reshape1 : Reshape  OutputDimensionality=Customize  OutputDimensions=[3,3]
  Vector Concatenate : Concatenate  NumInputs=9
  Vector Concatenate1 : Concatenate  NumInputs=9
  Zero : Constant  Value=0  OutDataTypeStr=Inherit: Inherit via back propagation
  Out1 : Outport
  wires:
  Reshape/1 -> MatrixMultiply1/1
  MatrixMultiply1/1 -> Out1/1  "rotation matrix"
  In1/1 -> Vector Concatenate1/4, Vector Concatenate1/2, Vector Concatenate/2  "amplitude of nonrothog 1"
  In2/1 -> Vector Concatenate/3, Vector Concatenate1/7, Vector Concatenate1/3  "amplitude of nonrothog 2"
  In3/1 -> Vector Concatenate1/8, Vector Concatenate1/6, Vector Concatenate/6  "amplitude of nonrothog 3"
  Vector Concatenate/1 -> Reshape/1
  Vector Concatenate1/1 -> Reshape1/1
  One/1 -> Vector Concatenate/5, Vector Concatenate/9, Vector Concatenate1/1, Vector Concatenate1/5, Vector Concatenate1/9, Vector Concatenate/1
  Zero/1 -> Vector Concatenate/8, Vector Concatenate/7, Vector Concatenate/4
  Reshape1/1 -> MatrixMultiply1/2

== system Project_sim/Sensors/Sun sensor/Noise ==
  In1 : Inport
  Add : Sum  Inputs=+++
  Discrete Transfer Fcn : DiscreteTransferFcn  LoadFcn=dspblkCoreblockFVToolHelper(gcbh,'load');  Numerator=[0.001*Ts_sun 0.001*Ts_sun]  Denominator=[2+0.001*Ts_sun 0.001*Ts_sun-2]
      settings: CopyFcn=dspblkCoreblockFVToolHelper(gcbh,'copy');  DeleteFcn=dspblkCoreblockFVToolHelper(gcbh,'close');  ModelCloseFcn=dspblkCoreblockFVToolHelper(gcbh,'close');  PreSaveFcn=dspblkCoreblockFVToolHelper(gcbh,'presave');  PostSaveFcn=dspblkCoreblockFVToolHelper(gcbh,'postsave');  CloseFcn=dspblkCoreblockFVToolHelper(gcbh,'close');
  Discrete Transfer Fcn1 : DiscreteTransferFcn  LoadFcn=dspblkCoreblockFVToolHelper(gcbh,'load');  Numerator=num_cz_sun  Denominator=den_cz_sun
      settings: CopyFcn=dspblkCoreblockFVToolHelper(gcbh,'copy');  DeleteFcn=dspblkCoreblockFVToolHelper(gcbh,'close');  ModelCloseFcn=dspblkCoreblockFVToolHelper(gcbh,'close');  PreSaveFcn=dspblkCoreblockFVToolHelper(gcbh,'presave');  PostSaveFcn=dspblkCoreblockFVToolHelper(gcbh,'postsave');  CloseFcn=dspblkCoreblockFVToolHelper(gcbh,'close');
  Product : Product
  Product1 : Product
  Product2 : Product
  Random Number : RandomNumber  Seed=randi(1e6)  SampleTime=Ts_sun
  Random Number4 : RandomNumber  Seed=randi(1e6)  SampleTime=Ts_sun
  Random Number5 : RandomNumber  Seed=randi(1e6)  SampleTime=Ts_sun
  Out1 : Outport
  wires:
  Product1/1 -> Discrete Transfer Fcn1/1
  Product/1 -> Discrete Transfer Fcn/1
  Product2/1 -> Add/3  "white noise"
  Discrete Transfer Fcn/1 -> Add/1  "brown noise"
  Discrete Transfer Fcn1/1 -> Add/2  "pink noise"
  Random Number/1 -> Product/2
  Add/1 -> Out1/1  "noise"
  In1/1 -> Product2/1, Product1/1, Product/1  "sigma"
  Random Number4/1 -> Product1/2
  Random Number5/1 -> Product2/2

== system Project_sim/Sensors/Sun sensor/Noise1 ==
  In1 : Inport
  Add : Sum  Inputs=+++
  Discrete Transfer Fcn : DiscreteTransferFcn  LoadFcn=dspblkCoreblockFVToolHelper(gcbh,'load');  Numerator=[0.001*Ts_sun 0.001*Ts_sun]  Denominator=[2+0.001*Ts_sun 0.001*Ts_sun-2]
      settings: CopyFcn=dspblkCoreblockFVToolHelper(gcbh,'copy');  DeleteFcn=dspblkCoreblockFVToolHelper(gcbh,'close');  ModelCloseFcn=dspblkCoreblockFVToolHelper(gcbh,'close');  PreSaveFcn=dspblkCoreblockFVToolHelper(gcbh,'presave');  PostSaveFcn=dspblkCoreblockFVToolHelper(gcbh,'postsave');  CloseFcn=dspblkCoreblockFVToolHelper(gcbh,'close');
  Discrete Transfer Fcn1 : DiscreteTransferFcn  LoadFcn=dspblkCoreblockFVToolHelper(gcbh,'load');  Numerator=num_cz_sun  Denominator=den_cz_sun
      settings: CopyFcn=dspblkCoreblockFVToolHelper(gcbh,'copy');  DeleteFcn=dspblkCoreblockFVToolHelper(gcbh,'close');  ModelCloseFcn=dspblkCoreblockFVToolHelper(gcbh,'close');  PreSaveFcn=dspblkCoreblockFVToolHelper(gcbh,'presave');  PostSaveFcn=dspblkCoreblockFVToolHelper(gcbh,'postsave');  CloseFcn=dspblkCoreblockFVToolHelper(gcbh,'close');
  Product : Product
  Product1 : Product
  Product2 : Product
  Random Number1 : RandomNumber  Seed=randi(1e6)  SampleTime=Ts_sun
  Random Number2 : RandomNumber  Seed=randi(1e6)  SampleTime=Ts_sun  VectorParams1D=off
  Random Number3 : RandomNumber  Seed=randi(1e6)  SampleTime=Ts_sun
  Out1 : Outport
  wires:
  Product1/1 -> Discrete Transfer Fcn1/1
  Product2/1 -> Add/3  "white noise"
  Discrete Transfer Fcn1/1 -> Add/2  "pink noise"
  Random Number2/1 -> Product/2
  Add/1 -> Out1/1  "noise"
  In1/1 -> Product2/1, Product1/1, Product/1  "sigma"
  Random Number1/1 -> Product1/2
  Random Number3/1 -> Product2/2
  Product/1 -> Discrete Transfer Fcn/1  "brown noise"
  Discrete Transfer Fcn/1 -> Add/1  "brown noise"

== system Project_sim/Sensors/Sun sensor/Noise2 ==
  In1 : Inport
  Add : Sum  Inputs=+++
  Discrete Transfer Fcn : DiscreteTransferFcn  LoadFcn=dspblkCoreblockFVToolHelper(gcbh,'load');  Numerator=[0.001*Ts_sun 0.001*Ts_sun]  Denominator=[2+0.001*Ts_sun 0.001*Ts_sun-2]
      settings: CopyFcn=dspblkCoreblockFVToolHelper(gcbh,'copy');  DeleteFcn=dspblkCoreblockFVToolHelper(gcbh,'close');  ModelCloseFcn=dspblkCoreblockFVToolHelper(gcbh,'close');  PreSaveFcn=dspblkCoreblockFVToolHelper(gcbh,'presave');  PostSaveFcn=dspblkCoreblockFVToolHelper(gcbh,'postsave');  CloseFcn=dspblkCoreblockFVToolHelper(gcbh,'close');
  Discrete Transfer Fcn1 : DiscreteTransferFcn  LoadFcn=dspblkCoreblockFVToolHelper(gcbh,'load');  Numerator=num_cz_sun  Denominator=den_cz_sun
      settings: CopyFcn=dspblkCoreblockFVToolHelper(gcbh,'copy');  DeleteFcn=dspblkCoreblockFVToolHelper(gcbh,'close');  ModelCloseFcn=dspblkCoreblockFVToolHelper(gcbh,'close');  PreSaveFcn=dspblkCoreblockFVToolHelper(gcbh,'presave');  PostSaveFcn=dspblkCoreblockFVToolHelper(gcbh,'postsave');  CloseFcn=dspblkCoreblockFVToolHelper(gcbh,'close');
  Product : Product
  Product1 : Product
  Product2 : Product
  Random Number1 : RandomNumber  Seed=randi(1e6)  SampleTime=Ts_sun
  Random Number2 : RandomNumber  Seed=randi(1e6)  SampleTime=Ts_sun
  Random Number3 : RandomNumber  Seed=randi(1e6)  SampleTime=Ts_sun
  Out1 : Outport
  wires:
  Product1/1 -> Discrete Transfer Fcn1/1
  Product/1 -> Discrete Transfer Fcn/1
  Product2/1 -> Add/3  "white noise"
  Discrete Transfer Fcn/1 -> Add/1  "brown noise"
  Random Number2/1 -> Product/2
  Add/1 -> Out1/1  "noise"
  In1/1 -> Product2/1, Product1/1, Product/1  "sigma"
  Random Number1/1 -> Product1/2
  Random Number3/1 -> Product2/2
  Discrete Transfer Fcn1/1 -> Add/2  "brown noise"

== system Project_sim/Sensors/Sun sensor/Precision ==
  In1 : Inport
  Acos1 : Trigonometry  Operator=acos
  Clock : Clock
  Constant3 : Constant  Value=[0; 0; 0]
  Dot Product1 : DotProduct  OutDataTypeStr=Inherit: Inherit via internal rule
  Latency1 : Delay  DelayLength=1
  Switch : Switch  Criteria=u2 > Threshold  Threshold=precision_sun  SaturateOnIntegerOverflow=off  InputSameDT=off
  Switch1 : Switch  Criteria=u2 ~= 0  SaturateOnIntegerOverflow=off  InputSameDT=off
  Out1 : Outport
  wires:
  Clock/1 -> Switch1/2
  Constant3/1 -> Switch1/3
  Latency1/1 -> Switch/3, Switch1/1
  Switch1/1 -> Dot Product1/1
  Switch/1 -> Out1/1, Latency1/1
  Acos1/1 -> Switch/2
  In1/1 -> Dot Product1/2, Switch/1
  Dot Product1/1 -> Acos1/1

== system Project_sim/Sensors/Sun sensor/Subsystem1 ==
  In1 : Inport
  In2 : Inport  Port=2
  In3 : Inport  Port=3
  A1 : Lib_rotation_matrix/A1  SystemSampleTime=-1  VariantActivationTime=update diagram  EmptyChoice=off  PassThrough=off  PassThroughVariantControl=(default)  EmptyChoiceVariantControl=(default)  AllowFlexibleInterface=on  Latency=0  AutoFrameSizeCalculation=off
  A2 : Lib_rotation_matrix/A2  SystemSampleTime=-1  VariantActivationTime=update diagram  EmptyChoice=off  PassThrough=off  PassThroughVariantControl=(default)  EmptyChoiceVariantControl=(default)  AllowFlexibleInterface=on  Latency=0  AutoFrameSizeCalculation=off
  A3 : Lib_rotation_matrix/A3  SystemSampleTime=-1  VariantActivationTime=update diagram  EmptyChoice=off  PassThrough=off  PassThroughVariantControl=(default)  EmptyChoiceVariantControl=(default)  AllowFlexibleInterface=on  Latency=0  AutoFrameSizeCalculation=off
  MatrixMultiply : Product  Multiplication=Matrix(*)
  MatrixMultiply1 : Product  Multiplication=Matrix(*)
  Out1 : Outport
  wires:
  MatrixMultiply/1 -> MatrixMultiply1/1
  In1/1 -> A1/1  "amplitude of rotation x"
  A3/1 -> MatrixMultiply1/2
  A1/1 -> MatrixMultiply/1
  MatrixMultiply1/1 -> Out1/1  "rotation matrix"
  A2/1 -> MatrixMultiply/2
  In2/1 -> A2/1  "amplitude of rotation y"
  In3/1 -> A3/1  "amplitude of rotation z"

== system Project_sim/Sensors/Sun sensor/Subsystem2 ==
  In1 : Inport
  In2 : Inport  Port=2
  In3 : Inport  Port=3
  A1 : Lib_rotation_matrix/A1  SystemSampleTime=-1  VariantActivationTime=update diagram  EmptyChoice=off  PassThrough=off  PassThroughVariantControl=(default)  EmptyChoiceVariantControl=(default)  AllowFlexibleInterface=on  Latency=0  AutoFrameSizeCalculation=off
  A2 : Lib_rotation_matrix/A2  SystemSampleTime=-1  VariantActivationTime=update diagram  EmptyChoice=off  PassThrough=off  PassThroughVariantControl=(default)  EmptyChoiceVariantControl=(default)  AllowFlexibleInterface=on  Latency=0  AutoFrameSizeCalculation=off
  A3 : Lib_rotation_matrix/A3  SystemSampleTime=-1  VariantActivationTime=update diagram  EmptyChoice=off  PassThrough=off  PassThroughVariantControl=(default)  EmptyChoiceVariantControl=(default)  AllowFlexibleInterface=on  Latency=0  AutoFrameSizeCalculation=off
  MatrixMultiply : Product  Multiplication=Matrix(*)
  MatrixMultiply1 : Product  Multiplication=Matrix(*)
  Out1 : Outport
  wires:
  MatrixMultiply/1 -> MatrixMultiply1/1
  A3/1 -> MatrixMultiply1/2
  A1/1 -> MatrixMultiply/1
  MatrixMultiply1/1 -> Out1/1  "rotation matrix"
  A2/1 -> MatrixMultiply/2
  In1/1 -> A1/1  "amplitude of misalignment x"
  In2/1 -> A2/1  "amplitude of misalignment y"
  In3/1 -> A3/1  "amplitude of misalignment z"

== system Project_sim/Reaction Wheels/Saturation/Max_torque(omega)/If Action Subsystem ==
  Action Port : ActionPort  ActionPortLabel=if(u2 <= u1 & u2 >= -u1)
  Constant : Constant  Value=RW.max_torque
  Out1 : Outport
  wires:
  Constant/1 -> Out1/1

== system Project_sim/Reaction Wheels/Saturation/Max_torque(omega)/If Action Subsystem1 ==
  In1 : Inport
  Action Port : ActionPort  ActionPortLabel=else
  Abs : Abs  SaturateOnIntegerOverflow=off
  Constant : Constant  Value=RW.max_torque_start_descending
  Constant1 : Constant  Value=RW.max_torque_descending_rate
  Constant2 : Constant  Value=RW.max_torque
  If : If  IfExpression=u1 >= 0
  If Action Subsystem : Subsystem  TreatAsAtomicUnit=on
  If Action Subsystem1 : Subsystem  TreatAsAtomicUnit=on
  Merge : Merge
  Product : Product
  Sum : Sum  Inputs=|+-
  Sum1 : Sum  Inputs=|++
  Out1 : Outport
  wires:
  In1/1 -> Abs/1
  Constant/1 -> Sum/2
  Sum/1 -> Product/1
  Constant1/1 -> Product/2
  Product/1 -> Sum1/1
  Constant2/1 -> Sum1/2
  Sum1/1 -> If Action Subsystem/1(In1), If/1
  If/1 -> If Action Subsystem/Action
  If/2 -> If Action Subsystem1/Action
  Merge/1 -> Out1/1
  If Action Subsystem1/1(Out1) -> Merge/2
  If Action Subsystem/1(Out1) -> Merge/1
  Abs/1 -> Sum/1

== system Project_sim/Reaction Wheels/Saturation/Max_torque(omega)1/If Action Subsystem ==
  Action Port : ActionPort  ActionPortLabel=if(u2 <= u1 & u2 >= -u1)
  Constant : Constant  Value=RW.max_torque
  Out1 : Outport
  wires:
  Constant/1 -> Out1/1

== system Project_sim/Reaction Wheels/Saturation/Max_torque(omega)1/If Action Subsystem1 ==
  In1 : Inport
  Action Port : ActionPort  ActionPortLabel=else
  Abs : Abs  SaturateOnIntegerOverflow=off
  Constant : Constant  Value=RW.max_torque_start_descending
  Constant1 : Constant  Value=RW.max_torque_descending_rate
  Constant2 : Constant  Value=RW.max_torque
  If : If  IfExpression=u1 >= 0
  If Action Subsystem : Subsystem  TreatAsAtomicUnit=on
  If Action Subsystem1 : Subsystem  TreatAsAtomicUnit=on
  Merge : Merge
  Product : Product
  Sum : Sum  Inputs=|+-
  Sum1 : Sum  Inputs=|++
  Out1 : Outport
  wires:
  In1/1 -> Abs/1
  Constant/1 -> Sum/2
  Sum/1 -> Product/1
  Constant1/1 -> Product/2
  Product/1 -> Sum1/1
  Constant2/1 -> Sum1/2
  Sum1/1 -> If Action Subsystem/1(In1), If/1
  If/1 -> If Action Subsystem/Action
  If/2 -> If Action Subsystem1/Action
  Merge/1 -> Out1/1
  If Action Subsystem1/1(Out1) -> Merge/2
  If Action Subsystem/1(Out1) -> Merge/1
  Abs/1 -> Sum/1

== system Project_sim/Reaction Wheels/Saturation/Max_torque(omega)2/If Action Subsystem ==
  Action Port : ActionPort  ActionPortLabel=if(u2 <= u1 & u2 >= -u1)
  Constant : Constant  Value=RW.max_torque
  Out1 : Outport
  wires:
  Constant/1 -> Out1/1

== system Project_sim/Reaction Wheels/Saturation/Max_torque(omega)2/If Action Subsystem1 ==
  In1 : Inport
  Action Port : ActionPort  ActionPortLabel=else
  Abs : Abs  SaturateOnIntegerOverflow=off
  Constant : Constant  Value=RW.max_torque_start_descending
  Constant1 : Constant  Value=RW.max_torque_descending_rate
  Constant2 : Constant  Value=RW.max_torque
  If : If  IfExpression=u1 >= 0
  If Action Subsystem : Subsystem  TreatAsAtomicUnit=on
  If Action Subsystem1 : Subsystem  TreatAsAtomicUnit=on
  Merge : Merge
  Product : Product
  Sum : Sum  Inputs=|+-
  Sum1 : Sum  Inputs=|++
  Out1 : Outport
  wires:
  In1/1 -> Abs/1
  Constant/1 -> Sum/2
  Sum/1 -> Product/1
  Constant1/1 -> Product/2
  Product/1 -> Sum1/1
  Constant2/1 -> Sum1/2
  Sum1/1 -> If Action Subsystem/1(In1), If/1
  If/1 -> If Action Subsystem/Action
  If/2 -> If Action Subsystem1/Action
  Merge/1 -> Out1/1
  If Action Subsystem1/1(Out1) -> Merge/2
  If Action Subsystem/1(Out1) -> Merge/1
  Abs/1 -> Sum/1

== system Project_sim/Reaction Wheels/Saturation/Max_torque(omega)/If Action Subsystem1/If Action Subsystem ==
  In1 : Inport
  Action Port : ActionPort  ActionPortLabel=if(u1 >= 0)
  Out1 : Outport
  wires:
  In1/1 -> Out1/1

== system Project_sim/Reaction Wheels/Saturation/Max_torque(omega)/If Action Subsystem1/If Action Subsystem1 ==
  Action Port : ActionPort  ActionPortLabel=else
  Zero : Constant  Value=0  OutDataTypeStr=Inherit: Inherit via back propagation
  Out1 : Outport
  wires:
  Zero/1 -> Out1/1

== system Project_sim/Reaction Wheels/Saturation/Max_torque(omega)1/If Action Subsystem1/If Action Subsystem ==
  In1 : Inport
  Action Port : ActionPort  ActionPortLabel=if(u1 >= 0)
  Out1 : Outport
  wires:
  In1/1 -> Out1/1

== system Project_sim/Reaction Wheels/Saturation/Max_torque(omega)1/If Action Subsystem1/If Action Subsystem1 ==
  Action Port : ActionPort  ActionPortLabel=else
  Zero : Constant  Value=0  OutDataTypeStr=Inherit: Inherit via back propagation
  Out1 : Outport
  wires:
  Zero/1 -> Out1/1

== system Project_sim/Reaction Wheels/Saturation/Max_torque(omega)2/If Action Subsystem1/If Action Subsystem ==
  In1 : Inport
  Action Port : ActionPort  ActionPortLabel=if(u1 >= 0)
  Out1 : Outport
  wires:
  In1/1 -> Out1/1

== system Project_sim/Reaction Wheels/Saturation/Max_torque(omega)2/If Action Subsystem1/If Action Subsystem1 ==
  Action Port : ActionPort  ActionPortLabel=else
  Zero : Constant  Value=0  OutDataTypeStr=Inherit: Inherit via back propagation
  Out1 : Outport
  wires:
  Zero/1 -> Out1/1

== matlab function Project_sim/Attitude determination/Attitude determination/MATLAB Function1 ==
  data: R input; q output
function q =max_eig(R)

[V,D]=eig(R);

eigenvalue=real(diag(D));
[~, index] = max(eigenvalue);
q=real(V(:,index));
